simulink model "Test"  (R2017a)
settings: Solver=VariableStepAuto  StartTime=0.0  StopTime=30  RelTol=1e-3
libraries: shared6dof x1, aerolibanim x1
settings Model: Creator=GusBus  LastModifiedBy=GusBus

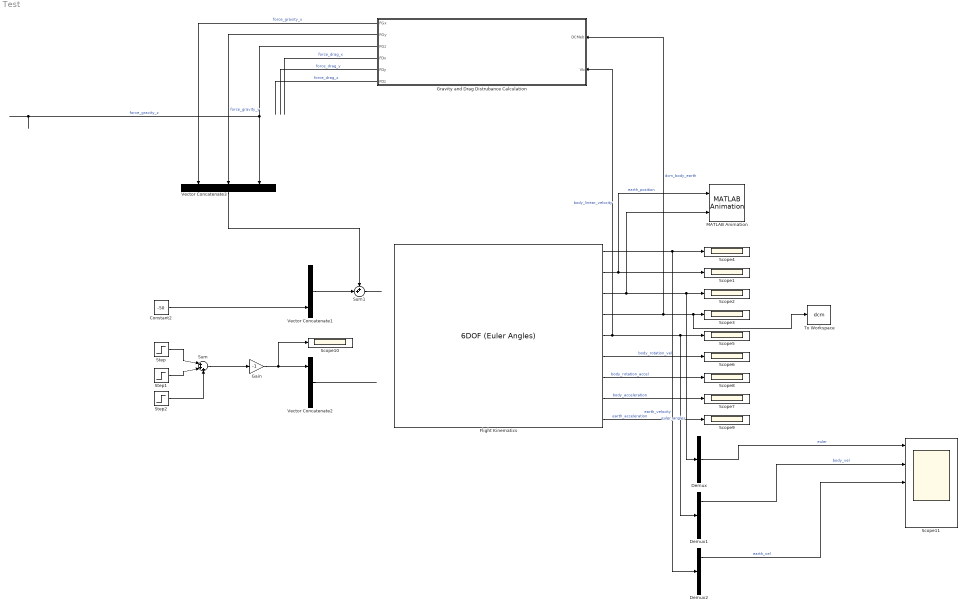
== system Test ==
  Constant2 : Constant  Value=-50
  Demux : Demux  Outputs=3
  Demux1 : Demux  Outputs=3
  Demux2 : Demux  Outputs=3
  Flight Kinematics : shared6dof/6DOF (Euler Angles)  units=Metric (MKS)  mtype=Fixed  rep=Euler Angles  xme_0=[0 0 0]  Vm_0=[0 0 0]  eul_0=[0.16 0 0]  pm_0=[0 0 0]  mass_0=3.352  mass_e=0.5  mass_f=2.0  inertia=[0.025028 0 0; 0 0.16926 0; 0 0 0.170197]  inertia_e=eye(3)  inertia_f=2*eye(3)  k_quat=1.0  vre_flag=on  abi_flag=on
  Gain : Gain  Gain=-1
  Gravity and Drag Distrubance Calculation : MATLAB Function  TreatAsAtomicUnit=on
  MATLAB Animation : aerolibanim/MATLAB Animation  Tag=Matlab Animation 6 DOF  Vehicles=1  Geometries='astredwedge.mat'  BoundingBoxCoordinates=[-50,50,-50,50,-50,50]  CameraOffset=[-150,0,0]  CameraViewAngle=3  SampleTime=0.2  FigurePosition=[2,42,958,981]
      settings: SourceProductName=Aerospace Blockset  SourceProductBaseCode=AE
  Scope{1..10} (10 alike) : Scope
  Scope11 : Scope  NumInputPorts=5
  Step : Step  After=-0.008  SampleTime=0
  Step1 : Step  Time=2  After=0.016  SampleTime=0
  Step2 : Step  Time=3  After=-0.008  SampleTime=0
  Sum : Sum  Inputs=|+++
  Sum1 : Sum  Inputs=++|
  To Workspace : ToWorkspace  VariableName=dcm  SampleTime=-1
      settings: Save2DSignal=2-D array (concatenate along first dimension)
  Vector Concatenate1 : Concatenate  NumInputs=3
  Vector Concatenate2 : Concatenate  NumInputs=3
  Vector Concatenate3 : Concatenate  NumInputs=3
  wires:
  Constant2/1 -> Vector Concatenate1/3
  Sum1/1 -> ?
  Vector Concatenate2/1 -> ?
  Flight Kinematics/1 -> Demux2/1, Scope4/1  "earth_velocity"
  Flight Kinematics/8 -> Scope7/1  "body_acceleration"
  Flight Kinematics/7 -> Scope8/1  "body_rotation_accel"
  Flight Kinematics/6 -> Scope6/1  "body_rotation_vel"
  Flight Kinematics/3 -> MATLAB Animation/2, Demux/1, Scope2/1  "euler_angles"
  Flight Kinematics/2 -> MATLAB Animation/1, Scope1/1  "earth_position"
  Flight Kinematics/9 -> Scope9/1  "earth_acceleration"
  Step/1 -> Sum/1
  Step1/1 -> Sum/2
  Step2/1 -> Sum/3
  Sum/1 -> Gain/1
  Demux/2 -> Scope11/1  "euler"
  Demux1/1 -> Scope11/2  "body_vel"
  Demux2/1 -> Scope11/3  "earth_vel"
  Gain/1 -> Vector Concatenate2/1, Scope10/1
  Flight Kinematics/4 -> Gravity and Drag Distrubance Calculation/1(DCMeb), To Workspace/1, Scope3/1  "dcm_body_earth"
  Flight Kinematics/5 -> Gravity and Drag Distrubance Calculation/2(Vb), Demux1/1, Scope5/1  "body_linear_velocity"
  Gravity and Drag Distrubance Calculation/3(FGz) -> Vector Concatenate3/3  "force_gravity_z"
  Gravity and Drag Distrubance Calculation/1(FGx) -> Vector Concatenate3/1  "force_gravity_x"
  Gravity and Drag Distrubance Calculation/4(FDx) -> ?  "force_drag_x"
  Gravity and Drag Distrubance Calculation/5(FDy) -> ?  "force_drag_y"
  Gravity and Drag Distrubance Calculation/6(FDz) -> ?  "force_drag_z"
  Gravity and Drag Distrubance Calculation/2(FGy) -> Vector Concatenate3/2  "force_gravity_y"
  Vector Concatenate3/1 -> Sum1/1
  Vector Concatenate1/1 -> Sum1/2

== matlab function Test/Gravity and Drag Distrubance Calculation ==
  data: DCMeb input; FGx output; Vb input; FGy output; FGz output; FDx output; FDy output; FDz output
function [FGx, FGy, FGz, FDx, FDy, FDz] = gravityDragCalculation(DCMeb, Vb)
%   Gravity and Drag Calculations
%   Inputs
%   DCMbe = Direct Cosine Matrix, from earth to body
%   Vb = Linear Velocity, body frame
%   Outputs
%   FGa = Force of gravity in the 'a' axis, body frame
%   FDa = Force of drag in the 'a' axis, body frame

%Gravity Constants
mass = 3.352;
gravityForce_earth = [0, 0, (9.81*mass)];

%Drag Constants
airDensity = 1.1644; %wikipedia air density at 30 degrees C
dragCoefficient = 1.0; %SLADe
surfaceArea = [0.1, 0.5, 0.7]; 
Vbx = Vb(1);
Vby = Vb(2);
Vbz = Vb(3);

%Gravity Calculations
FG = DCMeb*transpose(gravityForce_earth);
FGx = FG(1);
FGy = FG(2);
FGz = FG(3);

% FGx = 0;
% FGy = 0;
% FGz = 0;

%Drag Calculations
% FDx = 0.5 * airDensity * (Vbx^2) * dragCoefficient * surfaceArea(1);
% FDy = 0.5 * airDensity * (Vby^2) * dragCoefficient * surfaceArea(2);
% FDz = 0.5 * airDensity * (Vbz^2) * dragCoefficient * surfaceArea(3);

 FDx = 0;
 FDy = 0;
 FDz = 0;


%% Trying some stupid stuff
% if Vbx > 0.000000000001
%     FDx = 0;
%     FDy = 0;
%     FDz = 0;
% else 
%     FDx = 0.5 * airDensity * (Vbx^2) * dragCoefficient * surfaceArea(1);
%     FDy = 0.5 * airDensity * (Vby^2) * dragCoefficient * surfaceArea(2);
%     FDz = 0.5 * airDensity * (Vbz^2) * dragCoefficient * surfaceArea(3);
% end
